simulink model "LUT_liver_pancreas_30"  (R2023b)
settings: Solver=FixedStepAuto  StartTime=0  StopTime=10.1  FixedStep=Timegap  RelTol=1e-3
model workspace (MAT data in the model file):
  T1_input = 1.34
(part 3 of 3)

== system LUT_liver_pancreas_30/If Action Subsystem6/If Action Subsystem2/If Action Subsystem9/If Action Subsystem1 ==
  In1 : Inport
  Action Port : ActionPort  ActionPortLabel=elseif( u1 >= 1.915)
  LUT 1.92RR : Lookup_n-D  NumberOfTableDimensions=1  BreakpointsForDimension1=[455.9435;504.372;599.0655;693.4809;787.3591;880.8145;973.957;1066.868;1159.606;1252.211;1344.714;1437.137;1529.495;1621.801;1714.065;1806.294;1898.493]  Table=[400;500;600;700;800;900;1000;1100;1200;1300;1400;1500;1600;1700;1800;1900;2000]  InternalRulePriority=Speed  RndMeth=Simplest
  Out1 : Outport
  wires:
  In1/1 -> LUT 1.92RR/1
  LUT 1.92RR/1 -> Out1/1

== system LUT_liver_pancreas_30/If Action Subsystem6/If Action Subsystem2/If Action Subsystem9/If Action Subsystem10 ==
  In1 : Inport
  Action Port : ActionPort  ActionPortLabel=if(u1 >= 1.995)
  LUT 2.00RR : Lookup_n-D  NumberOfTableDimensions=1  BreakpointsForDimension1=[455.5145;504.0254;598.6788;693.0105;786.7675;880.0716;973.0395;1065.758;1158.289;1250.677;1342.954;1435.143;1527.263;1619.326;1711.343;1803.322;1895.269]  Table=[400;500;600;700;800;900;1000;1100;1200;1300;1400;1500;1600;1700;1800;1900;2000]  InternalRulePriority=Speed  RndMeth=Simplest
  Out1 : Outport
  wires:
  In1/1 -> LUT 2.00RR/1
  LUT 2.00RR/1 -> Out1/1

== system LUT_liver_pancreas_30/If Action Subsystem6/If Action Subsystem2/If Action Subsystem9/If Action Subsystem11 ==
  In1 : Inport
  Action Port : ActionPort  ActionPortLabel=elseif( u1 >= 1.905)
  LUT 1.91RR : Lookup_n-D  NumberOfTableDimensions=1  BreakpointsForDimension1=[455.9998;504.4183;599.1181;693.5456;787.4408;880.9168;974.083;1067.02;1159.785;1252.42;1344.953;1437.406;1529.796;1622.134;1714.431;1806.692;1898.925]  Table=[400;500;600;700;800;900;1000;1100;1200;1300;1400;1500;1600;1700;1800;1900;2000]  InternalRulePriority=Speed  RndMeth=Simplest
  Out1 : Outport
  wires:
  In1/1 -> LUT 1.91RR/1
  LUT 1.91RR/1 -> Out1/1

== system LUT_liver_pancreas_30/If Action Subsystem6/If Action Subsystem2/If Action Subsystem9/If Action Subsystem2 ==
  In1 : Inport
  Action Port : ActionPort  ActionPortLabel=else
  LUT 1.90RR : Lookup_n-D  NumberOfTableDimensions=1  BreakpointsForDimension1=[456.0568;504.4652;599.1718;693.6118;787.5242;881.0214;974.2116;1067.175;1159.968;1252.632;1345.195;1437.68;1530.102;1622.473;1714.802;1807.097;1899.364]  Table=[400;500;600;700;800;900;1000;1100;1200;1300;1400;1500;1600;1700;1800;1900;2000]  InternalRulePriority=Speed  RndMeth=Simplest
  Out1 : Outport
  wires:
  In1/1 -> LUT 1.90RR/1
  LUT 1.90RR/1 -> Out1/1

== system LUT_liver_pancreas_30/If Action Subsystem6/If Action Subsystem2/If Action Subsystem9/If Action Subsystem3 ==
  In1 : Inport
  Action Port : ActionPort  ActionPortLabel=elseif( u1 >= 1.925)
  LUT 1.93RR : Lookup_n-D  NumberOfTableDimensions=1  BreakpointsForDimension1=[455.8877;504.3265;599.0139;693.4176;787.2793;880.7143;973.8337;1066.719;1159.43;1252.007;1344.48;1436.872;1529.199;1621.474;1713.705;1805.902;1898.068]  Table=[400;500;600;700;800;900;1000;1100;1200;1300;1400;1500;1600;1700;1800;1900;2000]  InternalRulePriority=Speed  RndMeth=Simplest
  Out1 : Outport
  wires:
  In1/1 -> LUT 1.93RR/1
  LUT 1.93RR/1 -> Out1/1

== system LUT_liver_pancreas_30/If Action Subsystem6/If Action Subsystem2/If Action Subsystem9/If Action Subsystem4 ==
  In1 : Inport
  Action Port : ActionPort  ActionPortLabel=elseif( u1 >= 1.935)
  LUT 1.94RR : Lookup_n-D  NumberOfTableDimensions=1  BreakpointsForDimension1=[455.8326;504.2816;598.9633;693.3556;787.2012;880.6164;973.7129;1066.573;1159.257;1251.806;1344.25;1436.612;1528.908;1621.152;1713.351;1805.515;1897.649]  Table=[400;500;600;700;800;900;1000;1100;1200;1300;1400;1500;1600;1700;1800;1900;2000]  InternalRulePriority=Speed  RndMeth=Simplest
  Out1 : Outport
  wires:
  In1/1 -> LUT 1.94RR/1
  LUT 1.94RR/1 -> Out1/1

== system LUT_liver_pancreas_30/If Action Subsystem6/If Action Subsystem2/If Action Subsystem9/If Action Subsystem5 ==
  In1 : Inport
  Action Port : ActionPort  ActionPortLabel=elseif( u1 >= 1.955)
  LUT 1.96RR : Lookup_n-D  NumberOfTableDimensions=1  BreakpointsForDimension1=[455.7242;504.1937;598.8648;693.2355;787.0501;880.4267;973.4788;1066.29;1158.922;1251.415;1343.802;1436.105;1528.341;1620.523;1712.66;1804.761;1896.831]  Table=[400;500;600;700;800;900;1000;1100;1200;1300;1400;1500;1600;1700;1800;1900;2000]  InternalRulePriority=Speed  RndMeth=Simplest
  Out1 : Outport
  wires:
  In1/1 -> LUT 1.96RR/1
  LUT 1.96RR/1 -> Out1/1

== system LUT_liver_pancreas_30/If Action Subsystem6/If Action Subsystem2/If Action Subsystem9/If Action Subsystem6 ==
  In1 : Inport
  Action Port : ActionPort  ActionPortLabel=elseif( u1 >= 1.945)
  LUT 1.95RR : Lookup_n-D  NumberOfTableDimensions=1  BreakpointsForDimension1=[455.7781;504.2373;598.9136;693.2949;787.1248;880.5205;973.5946;1066.431;1159.088;1251.609;1344.024;1436.356;1528.622;1620.835;1713.003;1805.135;1897.237]  Table=[400;500;600;700;800;900;1000;1100;1200;1300;1400;1500;1600;1700;1800;1900;2000]  InternalRulePriority=Speed  RndMeth=Simplest
  Out1 : Outport
  wires:
  In1/1 -> LUT 1.95RR/1
  LUT 1.95RR/1 -> Out1/1

== system LUT_liver_pancreas_30/If Action Subsystem6/If Action Subsystem2/If Action Subsystem9/If Action Subsystem7 ==
  In1 : Inport
  Action Port : ActionPort  ActionPortLabel=elseif( u1 >= 1.965)
  LUT 1.97RR : Lookup_n-D  NumberOfTableDimensions=1  BreakpointsForDimension1=[455.6709;504.1507;598.817;693.1774;786.9771;880.335;973.3654;1066.153;1158.759;1251.225;1343.584;1435.858;1528.065;1620.216;1712.323;1804.393;1896.431]  Table=[400;500;600;700;800;900;1000;1100;1200;1300;1400;1500;1600;1700;1800;1900;2000]  InternalRulePriority=Speed  RndMeth=Simplest
  Out1 : Outport
  wires:
  In1/1 -> LUT 1.97RR/1
  LUT 1.97RR/1 -> Out1/1

== system LUT_liver_pancreas_30/If Action Subsystem6/If Action Subsystem2/If Action Subsystem9/If Action Subsystem8 ==
  In1 : Inport
  Action Port : ActionPort  ActionPortLabel=elseif( u1 >= 1.975)
  LUT 1.98RR : Lookup_n-D  NumberOfTableDimensions=1  BreakpointsForDimension1=[455.6182;504.1083;598.7701;693.1206;786.9056;880.2452;973.2545;1066.019;1158.599;1251.039;1343.37;1435.616;1527.793;1619.915;1711.991;1804.03;1896.038]  Table=[400;500;600;700;800;900;1000;1100;1200;1300;1400;1500;1600;1700;1800;1900;2000]  InternalRulePriority=Speed  RndMeth=Simplest
  Out1 : Outport
  wires:
  In1/1 -> LUT 1.98RR/1
  LUT 1.98RR/1 -> Out1/1

== system LUT_liver_pancreas_30/If Action Subsystem6/If Action Subsystem2/If Action Subsystem9/If Action Subsystem9 ==
  In1 : Inport
  Action Port : ActionPort  ActionPortLabel=elseif(u1 >= 1.985)
  LUT 1.99RR : Lookup_n-D  NumberOfTableDimensions=1  BreakpointsForDimension1=[455.5661;504.0666;598.724;693.065;786.8358;880.1575;973.1458;1065.887;1158.442;1250.856;1343.16;1435.377;1527.526;1619.618;1711.664;1803.673;1895.65]  Table=[400;500;600;700;800;900;1000;1100;1200;1300;1400;1500;1600;1700;1800;1900;2000]  InternalRulePriority=Speed  RndMeth=Simplest
  Out1 : Outport
  wires:
  In1/1 -> LUT 1.99RR/1
  LUT 1.99RR/1 -> Out1/1

== system LUT_liver_pancreas_30/If Action Subsystem6/If Action Subsystem3/If Action Subsystem5/If Action Subsystem1 ==
  In1 : Inport
  Action Port : ActionPort  ActionPortLabel=elseif( u1 >= 0.615)
  LUT 0.62RR : Lookup_n-D  NumberOfTableDimensions=1  BreakpointsForDimension1=[474.416;523.9877;628.6715;734.4256;840.4801;946.6435;1052.814;1158.916;1264.875;1370.592;1475.677;1583.601;1687.634;1792.249;1896.633;2000.682;2104.35]  Table=[400;500;600;700;800;900;1000;1100;1200;1300;1400;1500;1600;1700;1800;1900;2000]  InternalRulePriority=Speed  RndMeth=Simplest
  Out1 : Outport
  wires:
  In1/1 -> LUT 0.62RR/1
  LUT 0.62RR/1 -> Out1/1

== system LUT_liver_pancreas_30/If Action Subsystem6/If Action Subsystem3/If Action Subsystem5/If Action Subsystem10 ==
  In1 : Inport
  Action Port : ActionPort  ActionPortLabel=elseif( u1 >= 0.605)
  LUT 0.61RR : Lookup_n-D  NumberOfTableDimensions=1  BreakpointsForDimension1=[474.5062;524.0083;628.793;734.7015;840.9386;947.2965;1053.661;1159.944;1266.062;1371.887;1476.748;1584.656;1689.15;1793.79;1898.122;2002.06;2105.559]  Table=[400;500;600;700;800;900;1000;1100;1200;1300;1400;1500;1600;1700;1800;1900;2000]  InternalRulePriority=Speed  RndMeth=Simplest
  Out1 : Outport
  wires:
  In1/1 -> LUT 0.61RR/1
  LUT 0.61RR/1 -> Out1/1

== system LUT_liver_pancreas_30/If Action Subsystem6/If Action Subsystem3/If Action Subsystem5/If Action Subsystem2 ==
  In1 : Inport
  Action Port : ActionPort  ActionPortLabel=else
  LUT 0.6RR : Lookup_n-D  NumberOfTableDimensions=1  BreakpointsForDimension1=[474.5798;523.9872;628.8477;734.8914;841.2953;947.8326;1054.375;1160.822;1267.075;1372.968;1477.18;1585.674;1690.376;1794.983;1899.206;2002.969;2106.229]  Table=[400;500;600;700;800;900;1000;1100;1200;1300;1400;1500;1600;1700;1800;1900;2000]  InternalRulePriority=Speed  RndMeth=Simplest
  Out1 : Outport
  wires:
  In1/1 -> LUT 0.6RR/1
  LUT 0.6RR/1 -> Out1/1

== system LUT_liver_pancreas_30/If Action Subsystem6/If Action Subsystem3/If Action Subsystem5/If Action Subsystem3 ==
  In1 : Inport
  Action Port : ActionPort  ActionPortLabel=elseif( u1 >= 0.625)
  LUT 0.63RR : Lookup_n-D  NumberOfTableDimensions=1  BreakpointsForDimension1=[474.3098;523.9296;628.4913;734.0752;839.9339;945.8908;1051.855;1157.76;1263.543;1369.122;1474.249;1582.938;1685.883;1790.418;1894.805;1998.91;2102.686]  Table=[400;500;600;700;800;900;1000;1100;1200;1300;1400;1500;1600;1700;1800;1900;2000]  InternalRulePriority=Speed  RndMeth=Simplest
  Out1 : Outport
  wires:
  In1/1 -> LUT 0.63RR/1
  LUT 0.63RR/1 -> Out1/1

== system LUT_liver_pancreas_30/If Action Subsystem6/If Action Subsystem3/If Action Subsystem5/If Action Subsystem4 ==
  In1 : Inport
  Action Port : ActionPort  ActionPortLabel=elseif( u1 >= 0.635)
  LUT 0.64RR : Lookup_n-D  NumberOfTableDimensions=1  BreakpointsForDimension1=[474.1884;523.8379;628.2596;733.6604;839.313;945.0537;1050.802;1156.498;1262.089;1367.508;1472.584;1574.402;1683.952;1788.347;1892.694;1996.809;2100.64]  Table=[400;500;600;700;800;900;1000;1100;1200;1300;1400;1500;1600;1700;1800;1900;2000]  InternalRulePriority=Speed  RndMeth=Simplest
  Out1 : Outport
  wires:
  In1/1 -> LUT 0.64RR/1
  LUT 0.64RR/1 -> Out1/1

== system LUT_liver_pancreas_30/If Action Subsystem6/If Action Subsystem3/If Action Subsystem5/If Action Subsystem5 ==
  In1 : Inport
  Action Port : ActionPort  ActionPortLabel=elseif( u1 >= 0.655)
  LUT 0.66RR : Lookup_n-D  NumberOfTableDimensions=1  BreakpointsForDimension1=[473.9037;523.5678;627.668;732.6733;837.8912;943.1792;1048.473;1153.727;1258.902;1363.951;1468.782;1572.784;1679.806;1783.66;1887.816;1991.837;2095.654]  Table=[400;500;600;700;800;900;1000;1100;1200;1300;1400;1500;1600;1700;1800;1900;2000]  InternalRulePriority=Speed  RndMeth=Simplest
  Out1 : Outport
  wires:
  In1/1 -> LUT 0.66RR/1
  LUT 0.66RR/1 -> Out1/1

== system LUT_liver_pancreas_30/If Action Subsystem6/If Action Subsystem3/If Action Subsystem5/If Action Subsystem6 ==
  In1 : Inport
  Action Port : ActionPort  ActionPortLabel=elseif( u1 >= 0.645)
  LUT 0.65RR : Lookup_n-D  NumberOfTableDimensions=1  BreakpointsForDimension1=[474.0528;523.7162;627.9832;733.1903;838.6287;944.1458;1049.669;1155.148;1260.536;1365.777;1470.748;1574.214;1681.9;1786.081;1890.35;1994.435;2098.278]  Table=[400;500;600;700;800;900;1000;1100;1200;1300;1400;1500;1600;1700;1800;1900;2000]  InternalRulePriority=Speed  RndMeth=Simplest
  Out1 : Outport
  wires:
  In1/1 -> LUT 0.65RR/1
  LUT 0.65RR/1 -> Out1/1

== system LUT_liver_pancreas_30/If Action Subsystem6/If Action Subsystem3/If Action Subsystem5/If Action Subsystem7 ==
  In1 : Inport
  Action Port : ActionPort  ActionPortLabel=elseif( u1 >= 0.665)
  LUT 0.67RR : Lookup_n-D  NumberOfTableDimensions=1  BreakpointsForDimension1=[473.7423;523.3958;627.3195;732.1167;837.1095;942.1646;1047.224;1152.249;1257.204;1362.051;1466.718;1570.857;1677.824;1781.119;1885.13;1989.059;2092.817]  Table=[400;500;600;700;800;900;1000;1100;1200;1300;1400;1500;1600;1700;1800;1900;2000]  InternalRulePriority=Speed  RndMeth=Simplest
  Out1 : Outport
  wires:
  In1/1 -> LUT 0.67RR/1
  LUT 0.67RR/1 -> Out1/1

== system LUT_liver_pancreas_30/If Action Subsystem6/If Action Subsystem3/If Action Subsystem5/If Action Subsystem8 ==
  In1 : Inport
  Action Port : ActionPort  ActionPortLabel=elseif(u1 >= 0.675)
  LUT 0.68RR : Lookup_n-D  NumberOfTableDimensions=1  BreakpointsForDimension1=[473.5695;523.203;626.9426;731.527;836.2917;941.1114;1045.934;1150.726;1255.457;1360.093;1464.579;1568.697;1676.389;1778.492;1882.325;1986.137;2089.81]  Table=[400;500;600;700;800;900;1000;1100;1200;1300;1400;1500;1600;1700;1800;1900;2000]  InternalRulePriority=Speed  RndMeth=Simplest
  Out1 : Outport
  wires:
  In1/1 -> LUT 0.68RR/1
  LUT 0.68RR/1 -> Out1/1

== system LUT_liver_pancreas_30/If Action Subsystem6/If Action Subsystem3/If Action Subsystem5/If Action Subsystem9 ==
  In1 : Inport
  Action Port : ActionPort  ActionPortLabel=if(u1 >= 0.685)
  LUT 0.69RR : Lookup_n-D  NumberOfTableDimensions=1  BreakpointsForDimension1=[473.3863;522.992;626.5416;730.9101;835.4449;940.028;1044.613;1149.17;1253.672;1358.092;1462.386;1566.406;1667.106;1775.814;1879.429;1983.102;2086.667]  Table=[400;500;600;700;800;900;1000;1100;1200;1300;1400;1500;1600;1700;1800;1900;2000]  InternalRulePriority=Speed  RndMeth=Simplest
  Out1 : Outport
  wires:
  In1/1 -> LUT 0.69RR/1
  LUT 0.69RR/1 -> Out1/1

== system LUT_liver_pancreas_30/If Action Subsystem6/If Action Subsystem3/If Action Subsystem6/If Action Subsystem1 ==
  In1 : Inport
  Action Port : ActionPort  ActionPortLabel=elseif( u1 >= 0.515)
  LUT 0.52RR : Lookup_n-D  NumberOfTableDimensions=1  BreakpointsForDimension1=[474.5762;521.7393;625.6496;731.5358;838.1904;945.1164;1051.969;1158.437;1263.932;1371.564;1475.254;1578.61;1680.944;1782.085;1881.929;1980.397;2077.433]  Table=[400;500;600;700;800;900;1000;1100;1200;1300;1400;1500;1600;1700;1800;1900;2000]  InternalRulePriority=Speed  RndMeth=Simplest
  Out1 : Outport
  wires:
  In1/1 -> LUT 0.52RR/1
  LUT 0.52RR/1 -> Out1/1

== system LUT_liver_pancreas_30/If Action Subsystem6/If Action Subsystem3/If Action Subsystem6/If Action Subsystem10 ==
  In1 : Inport
  Action Port : ActionPort  ActionPortLabel=elseif( u1 >= 0.505)
  LUT 0.51RR : Lookup_n-D  NumberOfTableDimensions=1  BreakpointsForDimension1=[474.5205;521.1183;624.6064;730.2245;836.688;943.4438;1050.1;1156.292;1261.116;1368.302;1471.738;1574.405;1675.861;1775.944;1874.546;1971.588;2067.015]  Table=[400;500;600;700;800;900;1000;1100;1200;1300;1400;1500;1600;1700;1800;1900;2000]  InternalRulePriority=Speed  RndMeth=Simplest
  Out1 : Outport
  wires:
  In1/1 -> LUT 0.51RR/1
  LUT 0.51RR/1 -> Out1/1

== system LUT_liver_pancreas_30/If Action Subsystem6/If Action Subsystem3/If Action Subsystem6/If Action Subsystem2 ==
  In1 : Inport
  Action Port : ActionPort  ActionPortLabel=else
  LUT 0.50RR : Lookup_n-D  NumberOfTableDimensions=1  BreakpointsForDimension1=[474.463;520.4034;623.3708;728.6386;834.8363;941.3471;1047.726;1153.541;1257.231;1364.382;1467.272;1569.079;1669.469;1768.286;1865.417;1960.783;2054.337]  Table=[400;500;600;700;800;900;1000;1100;1200;1300;1400;1500;1600;1700;1800;1900;2000]  InternalRulePriority=Speed  RndMeth=Simplest
  Out1 : Outport
  wires:
  In1/1 -> LUT 0.50RR/1
  LUT 0.50RR/1 -> Out1/1

== system LUT_liver_pancreas_30/If Action Subsystem6/If Action Subsystem3/If Action Subsystem6/If Action Subsystem3 ==
  In1 : Inport
  Action Port : ActionPort  ActionPortLabel=elseif( u1 >= 0.525)
  LUT 0.53RR : Lookup_n-D  NumberOfTableDimensions=1  BreakpointsForDimension1=[474.6253;522.2718;626.5165;732.598;839.3776;946.4084;1053.386;1160.044;1265.963;1365.661;1477.938;1581.826;1684.873;1786.888;1887.77;1987.443;2085.85]  Table=[400;500;600;700;800;900;1000;1100;1200;1300;1400;1500;1600;1700;1800;1900;2000]  InternalRulePriority=Speed  RndMeth=Simplest
  Out1 : Outport
  wires:
  In1/1 -> LUT 0.53RR/1
  LUT 0.53RR/1 -> Out1/1

== system LUT_liver_pancreas_30/If Action Subsystem6/If Action Subsystem3/If Action Subsystem6/If Action Subsystem4 ==
  In1 : Inport
  Action Port : ActionPort  ActionPortLabel=elseif( u1 >= 0.535)
  LUT 0.54RR : Lookup_n-D  NumberOfTableDimensions=1  BreakpointsForDimension1=[474.6644;522.7214;627.2226;733.4352;840.282;947.3604;1054.402;1161.177;1267.368;1369.963;1479.904;1584.175;1687.789;1790.518;1892.259;1992.94;2092.504]  Table=[400;500;600;700;800;900;1000;1100;1200;1300;1400;1500;1600;1700;1800;1900;2000]  InternalRulePriority=Speed  RndMeth=Simplest
  Out1 : Outport
  wires:
  In1/1 -> LUT 0.54RR/1
  LUT 0.54RR/1 -> Out1/1

== system LUT_liver_pancreas_30/If Action Subsystem6/If Action Subsystem3/If Action Subsystem6/If Action Subsystem5 ==
  In1 : Inport
  Action Port : ActionPort  ActionPortLabel=elseif( u1 >= 0.555)
  LUT 0.56RR : Lookup_n-D  NumberOfTableDimensions=1  BreakpointsForDimension1=[474.702;523.3943;628.2103;734.5232;841.36;948.3917;1055.409;1162.239;1268.68;1373.96;1482.145;1586.707;1691.087;1794.838;1897.845;2000.041;2101.376]  Table=[400;500;600;700;800;900;1000;1100;1200;1300;1400;1500;1600;1700;1800;1900;2000]  InternalRulePriority=Speed  RndMeth=Simplest
  Out1 : Outport
  wires:
  In1/1 -> LUT 0.56RR/1
  LUT 0.56RR/1 -> Out1/1

== system LUT_liver_pancreas_30/If Action Subsystem6/If Action Subsystem3/If Action Subsystem6/If Action Subsystem6 ==
  In1 : Inport
  Action Port : ActionPort  ActionPortLabel=elseif( u1 >= 0.545)
  LUT 0.55RR : Lookup_n-D  NumberOfTableDimensions=1  BreakpointsForDimension1=[474.6906;523.0937;627.7826;734.0699;840.9336;948.01;1055.062;1161.891;1268.247;1372.673;1481.264;1585.769;1689.822;1793.124;1895.566;1997.081;2097.613]  Table=[400;500;600;700;800;900;1000;1100;1200;1300;1400;1500;1600;1700;1800;1900;2000]  InternalRulePriority=Speed  RndMeth=Simplest
  Out1 : Outport
  wires:
  In1/1 -> LUT 0.55RR/1
  LUT 0.55RR/1 -> Out1/1

== system LUT_liver_pancreas_30/If Action Subsystem6/If Action Subsystem3/If Action Subsystem6/If Action Subsystem7 ==
  In1 : Inport
  Action Port : ActionPort  ActionPortLabel=elseif( u1 >= 0.565)
  LUT 0.57RR : Lookup_n-D  NumberOfTableDimensions=1  BreakpointsForDimension1=[474.6972;523.6287;628.519;734.8148;841.587;948.5373;1055.481;1162.266;1268.728;1374.402;1482.732;1587.083;1691.687;1795.78;1899.232;2001.978;2103.969]  Table=[400;500;600;700;800;900;1000;1100;1200;1300;1400;1500;1600;1700;1800;1900;2000]  InternalRulePriority=Speed  RndMeth=Simplest
  Out1 : Outport
  wires:
  In1/1 -> LUT 0.57RR/1
  LUT 0.57RR/1 -> Out1/1

== system LUT_liver_pancreas_30/If Action Subsystem6/If Action Subsystem3/If Action Subsystem6/If Action Subsystem8 ==
  In1 : Inport
  Action Port : ActionPort  ActionPortLabel=elseif(u1 >= 0.575)
  LUT 0.58RR : Lookup_n-D  NumberOfTableDimensions=1  BreakpointsForDimension1=[474.6754;523.8022;628.7207;734.9626;841.638;948.4755;1055.312;1162.015;1268.446;1374.298;1473.533;1586.981;1691.715;1796.057;1899.852;2003.032;2105.551]  Table=[400;500;600;700;800;900;1000;1100;1200;1300;1400;1500;1600;1700;1800;1900;2000]  InternalRulePriority=Speed  RndMeth=Simplest
  Out1 : Outport
  wires:
  In1/1 -> LUT 0.58RR/1
  LUT 0.58RR/1 -> Out1/1

== system LUT_liver_pancreas_30/If Action Subsystem6/If Action Subsystem3/If Action Subsystem6/If Action Subsystem9 ==
  In1 : Inport
  Action Port : ActionPort  ActionPortLabel=if(u1 >= 0.585)
  LUT 0.59RR : Lookup_n-D  NumberOfTableDimensions=1  BreakpointsForDimension1=[474.6363;523.9201;628.8268;734.9831;841.5343;948.2328;1054.934;1161.522;1267.881;1373.792;1476.295;1586.484;1691.253;1795.763;1899.811;2003.325;2106.263]  Table=[400;500;600;700;800;900;1000;1100;1200;1300;1400;1500;1600;1700;1800;1900;2000]  InternalRulePriority=Speed  RndMeth=Simplest
  Out1 : Outport
  wires:
  In1/1 -> LUT 0.59RR/1
  LUT 0.59RR/1 -> Out1/1

== system LUT_liver_pancreas_30/If Action Subsystem6/If Action Subsystem3/If Action Subsystem7/If Action Subsystem1 ==
  In1 : Inport
  Action Port : ActionPort  ActionPortLabel=elseif( u1 >= 0.715)
  LUT 0.72RR : Lookup_n-D  NumberOfTableDimensions=1  BreakpointsForDimension1=[472.7837;522.2728;625.232;728.945;832.7895;936.6649;1040.537;1144.387;1248.198;1351.952;1455.625;1559.161;1662.226;1768.021;1870.441;1973.584;2076.721]  Table=[400;500;600;700;800;900;1000;1100;1200;1300;1400;1500;1600;1700;1800;1900;2000]  InternalRulePriority=Speed  RndMeth=Simplest
  Out1 : Outport
  wires:
  In1/1 -> LUT 0.72RR/1
  LUT 0.72RR/1 -> Out1/1

== system LUT_liver_pancreas_30/If Action Subsystem6/If Action Subsystem3/If Action Subsystem7/If Action Subsystem10 ==
  In1 : Inport
  Action Port : ActionPort  ActionPortLabel=elseif( u1 >= 0.705)
  LUT 0.71RR : Lookup_n-D  NumberOfTableDimensions=1  BreakpointsForDimension1=[472.9925;522.5248;625.683;729.6147;833.6886;937.7988;1041.908;1145.992;1250.034;1354.012;1457.896;1561.613;1664.565;1770.484;1873.466;1976.804;2080.098]  Table=[400;500;600;700;800;900;1000;1100;1200;1300;1400;1500;1600;1700;1800;1900;2000]  InternalRulePriority=Speed  RndMeth=Simplest
  Out1 : Outport
  wires:
  In1/1 -> LUT 0.71RR/1
  LUT 0.71RR/1 -> Out1/1

== system LUT_liver_pancreas_30/If Action Subsystem6/If Action Subsystem3/If Action Subsystem7/If Action Subsystem2 ==
  In1 : Inport
  Action Port : ActionPort  ActionPortLabel=else
  LUT 0.70RR : Lookup_n-D  NumberOfTableDimensions=1  BreakpointsForDimension1=[473.1936;522.7652;626.1206;730.2711;834.5754;938.9217;1043.268;1147.589;1251.861;1356.062;1460.154;1564.034;1666.473;1773.124;1876.469;1979.983;2083.421]  Table=[400;500;600;700;800;900;1000;1100;1200;1300;1400;1500;1600;1700;1800;1900;2000]  InternalRulePriority=Speed  RndMeth=Simplest
  Out1 : Outport
  wires:
  In1/1 -> LUT 0.70RR/1
  LUT 0.70RR/1 -> Out1/1

== system LUT_liver_pancreas_30/If Action Subsystem6/If Action Subsystem3/If Action Subsystem7/If Action Subsystem3 ==
  In1 : Inport
  Action Port : ActionPort  ActionPortLabel=elseif( u1 >= 0.725)
  LUT 0.73RR : Lookup_n-D  NumberOfTableDimensions=1  BreakpointsForDimension1=[472.5683;522.011;624.7704;728.2654;831.8822;935.5249;1039.163;1142.779;1246.36;1349.89;1453.35;1556.696;1659.72;1766.121;1867.415;1970.342;2073.311]  Table=[400;500;600;700;800;900;1000;1100;1200;1300;1400;1500;1600;1700;1800;1900;2000]  InternalRulePriority=Speed  RndMeth=Simplest
  Out1 : Outport
  wires:
  In1/1 -> LUT 0.73RR/1
  LUT 0.73RR/1 -> Out1/1

== system LUT_liver_pancreas_30/If Action Subsystem6/If Action Subsystem3/If Action Subsystem7/If Action Subsystem4 ==
  In1 : Inport
  Action Port : ActionPort  ActionPortLabel=elseif( u1 >= 0.735)
  LUT 0.74RR : Lookup_n-D  NumberOfTableDimensions=1  BreakpointsForDimension1=[472.3471;521.741;624.3008;727.5792;830.9705;934.3829;1037.789;1141.174;1244.526;1347.833;1451.079;1554.227;1657.143;1766.068;1864.407;1967.093;2069.882]  Table=[400;500;600;700;800;900;1000;1100;1200;1300;1400;1500;1600;1700;1800;1900;2000]  InternalRulePriority=Speed  RndMeth=Simplest
  Out1 : Outport
  wires:
  In1/1 -> LUT 0.74RR/1
  LUT 0.74RR/1 -> Out1/1

== system LUT_liver_pancreas_30/If Action Subsystem6/If Action Subsystem3/If Action Subsystem7/If Action Subsystem5 ==
  In1 : Inport
  Action Port : ActionPort  ActionPortLabel=elseif( u1 >= 0.755)
  LUT 0.76RR : Lookup_n-D  NumberOfTableDimensions=1  BreakpointsForDimension1=[471.8903;521.182;623.3456;726.1977;829.1462;932.1073;1035.058;1137.989;1240.892;1343.757;1446.574;1549.319;1651.925;1753.767;1858.578;1960.627;2063.029]  Table=[400;500;600;700;800;900;1000;1100;1200;1300;1400;1500;1600;1700;1800;1900;2000]  InternalRulePriority=Speed  RndMeth=Simplest
  Out1 : Outport
  wires:
  In1/1 -> LUT 0.76RR/1
  LUT 0.76RR/1 -> Out1/1

== system LUT_liver_pancreas_30/If Action Subsystem6/If Action Subsystem3/If Action Subsystem7/If Action Subsystem6 ==
  In1 : Inport
  Action Port : ActionPort  ActionPortLabel=elseif( u1 >= 0.745)
  LUT 0.75RR : Lookup_n-D  NumberOfTableDimensions=1  BreakpointsForDimension1=[472.1208;521.4642;623.8252;726.8892;830.0576;933.2427;1036.42;1139.576;1242.702;1345.787;1448.818;1551.766;1654.537;1755.796;1861.447;1963.851;2066.451]  Table=[400;500;600;700;800;900;1000;1100;1200;1300;1400;1500;1600;1700;1800;1900;2000]  InternalRulePriority=Speed  RndMeth=Simplest
  Out1 : Outport
  wires:
  In1/1 -> LUT 0.75RR/1
  LUT 0.75RR/1 -> Out1/1

== system LUT_liver_pancreas_30/If Action Subsystem6/If Action Subsystem3/If Action Subsystem7/If Action Subsystem7 ==
  In1 : Inport
  Action Port : ActionPort  ActionPortLabel=elseif( u1 >= 0.765)
  LUT 0.77RR : Lookup_n-D  NumberOfTableDimensions=1  BreakpointsForDimension1=[471.6561;520.8957;622.8639;725.5068;828.2389;930.9794;1033.708;1136.417;1239.099;1341.746;1444.35;1546.892;1649.322;1751.296;1855.899;1957.433;2059.627]  Table=[400;500;600;700;800;900;1000;1100;1200;1300;1400;1500;1600;1700;1800;1900;2000]  InternalRulePriority=Speed  RndMeth=Simplest
  Out1 : Outport
  wires:
  In1/1 -> LUT 0.77RR/1
  LUT 0.77RR/1 -> Out1/1

== system LUT_liver_pancreas_30/If Action Subsystem6/If Action Subsystem3/If Action Subsystem7/If Action Subsystem8 ==
  In1 : Inport
  Action Port : ActionPort  ActionPortLabel=elseif(u1 >= 0.775)
  LUT 0.78RR : Lookup_n-D  NumberOfTableDimensions=1  BreakpointsForDimension1=[471.4191;520.6062;622.3814;724.8183;827.3375;929.8614;1032.372;1134.862;1237.326;1339.759;1442.152;1544.491;1646.737;1748.681;1853.716;1954.282;2056.254]  Table=[400;500;600;700;800;900;1000;1100;1200;1300;1400;1500;1600;1700;1800;1900;2000]  InternalRulePriority=Speed  RndMeth=Simplest
  Out1 : Outport
  wires:
  In1/1 -> LUT 0.78RR/1
  LUT 0.78RR/1 -> Out1/1

== system LUT_liver_pancreas_30/If Action Subsystem6/If Action Subsystem3/If Action Subsystem7/If Action Subsystem9 ==
  In1 : Inport
  Action Port : ActionPort  ActionPortLabel=if(u1 >= 0.785)
  LUT 0.79RR : Lookup_n-D  NumberOfTableDimensions=1  BreakpointsForDimension1=[471.1797;520.3146;621.8995;724.1339;826.444;928.7551;1031.051;1133.326;1235.576;1337.797;1439.982;1542.119;1644.179;1746.023;1853.155;1951.185;2052.917]  Table=[400;500;600;700;800;900;1000;1100;1200;1300;1400;1500;1600;1700;1800;1900;2000]  InternalRulePriority=Speed  RndMeth=Simplest
  Out1 : Outport
  wires:
  In1/1 -> LUT 0.79RR/1
  LUT 0.79RR/1 -> Out1/1

== system LUT_liver_pancreas_30/If Action Subsystem6/If Action Subsystem3/If Action Subsystem8/If Action Subsystem1 ==
  In1 : Inport
  Action Port : ActionPort  ActionPortLabel=elseif( u1 >= 0.815)
  LUT 0.82RR : Lookup_n-D  NumberOfTableDimensions=1  BreakpointsForDimension1=[470.4531;519.4351;620.4683;722.1174;823.8242;925.5214;1027.198;1128.852;1230.483;1332.089;1433.666;1535.209;1636.702;1738.096;1839.013;1942.508;2043.189]  Table=[400;500;600;700;800;900;1000;1100;1200;1300;1400;1500;1600;1700;1800;1900;2000]  InternalRulePriority=Speed  RndMeth=Simplest
  Out1 : Outport
  wires:
  In1/1 -> LUT 0.82RR/1
  LUT 0.82RR/1 -> Out1/1

== system LUT_liver_pancreas_30/If Action Subsystem6/If Action Subsystem3/If Action Subsystem8/If Action Subsystem10 ==
  In1 : Inport
  Action Port : ActionPort  ActionPortLabel=elseif( u1 >= 0.805)
  LUT 0.81RR : Lookup_n-D  NumberOfTableDimensions=1  BreakpointsForDimension1=[470.6962;519.7283;620.942;722.7824;824.6862;926.5838;1028.463;1130.32;1232.153;1333.96;1435.737;1537.476;1639.158;1740.714;1841.442;1945.245;2046.378]  Table=[400;500;600;700;800;900;1000;1100;1200;1300;1400;1500;1600;1700;1800;1900;2000]  InternalRulePriority=Speed  RndMeth=Simplest
  Out1 : Outport
  wires:
  In1/1 -> LUT 0.81RR/1
  LUT 0.81RR/1 -> Out1/1

== system LUT_liver_pancreas_30/If Action Subsystem6/If Action Subsystem3/If Action Subsystem8/If Action Subsystem2 ==
  In1 : Inport
  Action Port : ActionPort  ActionPortLabel=else
  LUT 0.80RR : Lookup_n-D  NumberOfTableDimensions=1  BreakpointsForDimension1=[470.9386;520.0217;621.4194;723.4549;825.5598;927.6621;1029.747;1131.811;1233.851;1335.864;1437.843;1539.78;1641.651;1743.36;1843.325;1948.162;2049.623]  Table=[400;500;600;700;800;900;1000;1100;1200;1300;1400;1500;1600;1700;1800;1900;2000]  InternalRulePriority=Speed  RndMeth=Simplest
  Out1 : Outport
  wires:
  In1/1 -> LUT 0.80RR/1
  LUT 0.80RR/1 -> Out1/1

== system LUT_liver_pancreas_30/If Action Subsystem6/If Action Subsystem3/If Action Subsystem8/If Action Subsystem3 ==
  In1 : Inport
  Action Port : ActionPort  ActionPortLabel=elseif( u1 >= 0.825)
  LUT 0.83RR : Lookup_n-D  NumberOfTableDimensions=1  BreakpointsForDimension1=[470.2097;519.1426;619.999;721.4608;822.9747;924.4756;1025.954;1127.409;1228.841;1330.25;1431.631;1532.981;1634.287;1735.512;1836.429;1940.169;2040.062]  Table=[400;500;600;700;800;900;1000;1100;1200;1300;1400;1500;1600;1700;1800;1900;2000]  InternalRulePriority=Speed  RndMeth=Simplest
  Out1 : Outport
  wires:
  In1/1 -> LUT 0.83RR/1
  LUT 0.83RR/1 -> Out1/1

== system LUT_liver_pancreas_30/If Action Subsystem6/If Action Subsystem3/If Action Subsystem8/If Action Subsystem4 ==
  In1 : Inport
  Action Port : ActionPort  ActionPortLabel=elseif( u1 >= 0.835)
  LUT 0.84RR : Lookup_n-D  NumberOfTableDimensions=1  BreakpointsForDimension1=[469.9663;518.8514;619.5346;720.8133;822.1384;923.4473;1024.732;1125.992;1227.23;1328.444;1429.633;1530.793;1631.914;1732.967;1833.806;1939.076;2037.006]  Table=[400;500;600;700;800;900;1000;1100;1200;1300;1400;1500;1600;1700;1800;1900;2000]  InternalRulePriority=Speed  RndMeth=Simplest
  Out1 : Outport
  wires:
  In1/1 -> LUT 0.84RR/1
  LUT 0.84RR/1 -> Out1/1

== system LUT_liver_pancreas_30/If Action Subsystem6/If Action Subsystem3/If Action Subsystem8/If Action Subsystem5 ==
  In1 : Inport
  Action Port : ActionPort  ActionPortLabel=elseif( u1 >= 0.855)
  LUT 0.86RR : Lookup_n-D  NumberOfTableDimensions=1  BreakpointsForDimension1=[469.4814;518.2747;618.6232;719.5475;820.5076;921.4451;1022.355;1123.238;1224.098;1324.935;1425.75;1526.54;1627.298;1728.006;1828.594;1928.211;2031.167]  Table=[400;500;600;700;800;900;1000;1100;1200;1300;1400;1500;1600;1700;1800;1900;2000]  InternalRulePriority=Speed  RndMeth=Simplest
  Out1 : Outport
  wires:
  In1/1 -> LUT 0.86RR/1
  LUT 0.86RR/1 -> Out1/1

== system LUT_liver_pancreas_30/If Action Subsystem6/If Action Subsystem3/If Action Subsystem8/If Action Subsystem6 ==
  In1 : Inport
  Action Port : ActionPort  ActionPortLabel=elseif( u1 >= 0.845)
  LUT 0.85RR : Lookup_n-D  NumberOfTableDimensions=1  BreakpointsForDimension1=[469.7235;518.5619;619.0759;720.1753;821.3159;922.437;1023.532;1124.602;1225.649;1326.672;1427.673;1528.646;1629.584;1730.465;1831.188;1941.317;2034.033]  Table=[400;500;600;700;800;900;1000;1100;1200;1300;1400;1500;1600;1700;1800;1900;2000]  InternalRulePriority=Speed  RndMeth=Simplest
  Out1 : Outport
  wires:
  In1/1 -> LUT 0.85RR/1
  LUT 0.85RR/1 -> Out1/1

== system LUT_liver_pancreas_30/If Action Subsystem6/If Action Subsystem3/If Action Subsystem8/If Action Subsystem7 ==
  In1 : Inport
  Action Port : ActionPort  ActionPortLabel=elseif( u1 >= 0.865)
  LUT 0.87RR : Lookup_n-D  NumberOfTableDimensions=1  BreakpointsForDimension1=[469.2404;517.99;618.1768;718.93;819.7139;920.4719;1021.2;1121.901;1222.578;1323.233;1423.866;1524.475;1625.056;1725.593;1826.035;1925.946;2028.461]  Table=[400;500;600;700;800;900;1000;1100;1200;1300;1400;1500;1600;1700;1800;1900;2000]  InternalRulePriority=Speed  RndMeth=Simplest
  Out1 : Outport
  wires:
  In1/1 -> LUT 0.87RR/1
  LUT 0.87RR/1 -> Out1/1

== system LUT_liver_pancreas_30/If Action Subsystem6/If Action Subsystem3/If Action Subsystem8/If Action Subsystem8 ==
  In1 : Inport
  Action Port : ActionPort  ActionPortLabel=elseif(u1 >= 0.875)
  LUT 0.88RR : Lookup_n-D  NumberOfTableDimensions=1  BreakpointsForDimension1=[469.0007;517.7081;617.7372;718.3234;818.935;919.5176;1020.068;1120.591;1221.089;1321.565;1422.02;1522.452;1622.858;1723.226;1823.517;1923.475;2026.064]  Table=[400;500;600;700;800;900;1000;1100;1200;1300;1400;1500;1600;1700;1800;1900;2000]  InternalRulePriority=Speed  RndMeth=Simplest
  Out1 : Outport
  wires:
  In1/1 -> LUT 0.88RR/1
  LUT 0.88RR/1 -> Out1/1

== system LUT_liver_pancreas_30/If Action Subsystem6/If Action Subsystem3/If Action Subsystem8/If Action Subsystem9 ==
  In1 : Inport
  Action Port : ActionPort  ActionPortLabel=if(u1 >= 0.885)
  LUT 0.89RR : Lookup_n-D  NumberOfTableDimensions=1  BreakpointsForDimension1=[468.7627;517.4293;617.3046;717.7277;818.171;918.5823;1018.96;1119.308;1219.631;1319.932;1420.212;1520.471;1620.705;1720.905;1821.042;1920.953;2024.538]  Table=[400;500;600;700;800;900;1000;1100;1200;1300;1400;1500;1600;1700;1800;1900;2000]  InternalRulePriority=Speed  RndMeth=Simplest
  Out1 : Outport
  wires:
  In1/1 -> LUT 0.89RR/1
  LUT 0.89RR/1 -> Out1/1

== system LUT_liver_pancreas_30/If Action Subsystem6/If Action Subsystem3/If Action Subsystem9/If Action Subsystem1 ==
  In1 : Inport
  Action Port : ActionPort  ActionPortLabel=elseif( u1 >= 0.915)
  LUT 0.92RR : Lookup_n-D  NumberOfTableDimensions=1  BreakpointsForDimension1=[468.06;516.6138;616.0504;716.0075;815.9697;915.8904;1015.771;1115.619;1215.44;1315.238;1415.016;1514.774;1614.512;1714.224;1813.897;1913.473;2012.422]  Table=[400;500;600;700;800;900;1000;1100;1200;1300;1400;1500;1600;1700;1800;1900;2000]  InternalRulePriority=Speed  RndMeth=Simplest
  Out1 : Outport
  wires:
  In1/1 -> LUT 0.92RR/1
  LUT 0.92RR/1 -> Out1/1

== system LUT_liver_pancreas_30/If Action Subsystem6/If Action Subsystem3/If Action Subsystem9/If Action Subsystem10 ==
  In1 : Inport
  Action Port : ActionPort  ActionPortLabel=elseif( u1 >= 0.905)
  LUT 0.91RR : Lookup_n-D  NumberOfTableDimensions=1  BreakpointsForDimension1=[468.2921;516.882;616.4611;716.5697;816.6884;916.7688;1016.811;1116.822;1216.807;1316.769;1416.711;1516.632;1616.532;1716.405;1816.231;1915.935;2014.415]  Table=[400;500;600;700;800;900;1000;1100;1200;1300;1400;1500;1600;1700;1800;1900;2000]  InternalRulePriority=Speed  RndMeth=Simplest
  Out1 : Outport
  wires:
  In1/1 -> LUT 0.91RR/1
  LUT 0.91RR/1 -> Out1/1

== system LUT_liver_pancreas_30/If Action Subsystem6/If Action Subsystem3/If Action Subsystem9/If Action Subsystem2 ==
  In1 : Inport
  Action Port : ActionPort  ActionPortLabel=else
  LUT 0.90RR : Lookup_n-D  NumberOfTableDimensions=1  BreakpointsForDimension1=[468.5264;517.1539;616.8792;717.1431;817.4222;917.6661;1017.874;1118.052;1218.204;1318.333;1418.443;1518.531;1618.597;1718.632;1818.613;1918.432;2025.833]  Table=[400;500;600;700;800;900;1000;1100;1200;1300;1400;1500;1600;1700;1800;1900;2000]  InternalRulePriority=Speed  RndMeth=Simplest
  Out1 : Outport
  wires:
  In1/1 -> LUT 0.90RR/1
  LUT 0.90RR/1 -> Out1/1

== system LUT_liver_pancreas_30/If Action Subsystem6/If Action Subsystem3/If Action Subsystem9/If Action Subsystem3 ==
  In1 : Inport
  Action Port : ActionPort  ActionPortLabel=elseif( u1 >= 0.925)
  LUT 0.93RR : Lookup_n-D  NumberOfTableDimensions=1  BreakpointsForDimension1=[467.8302;516.3494;615.6473;715.4567;815.2661;915.0307;1014.753;1114.442;1214.102;1313.74;1413.357;1512.956;1612.534;1712.089;1811.609;1911.052;2010.117]  Table=[400;500;600;700;800;900;1000;1100;1200;1300;1400;1500;1600;1700;1800;1900;2000]  InternalRulePriority=Speed  RndMeth=Simplest
  Out1 : Outport
  wires:
  In1/1 -> LUT 0.93RR/1
  LUT 0.93RR/1 -> Out1/1

== system LUT_liver_pancreas_30/If Action Subsystem6/If Action Subsystem3/If Action Subsystem9/If Action Subsystem4 ==
  In1 : Inport
  Action Port : ActionPort  ActionPortLabel=elseif( u1 >= 0.935)
  LUT 0.94RR : Lookup_n-D  NumberOfTableDimensions=1  BreakpointsForDimension1=[467.6029;516.089;615.2518;714.9171;814.5773;914.1896;1013.758;1113.29;1212.794;1312.275;1411.735;1511.177;1610.599;1710;1809.369;1908.675;2007.731]  Table=[400;500;600;700;800;900;1000;1100;1200;1300;1400;1500;1600;1700;1800;1900;2000]  InternalRulePriority=Speed  RndMeth=Simplest
  Out1 : Outport
  wires:
  In1/1 -> LUT 0.94RR/1
  LUT 0.94RR/1 -> Out1/1

== system LUT_liver_pancreas_30/If Action Subsystem6/If Action Subsystem3/If Action Subsystem9/If Action Subsystem5 ==
  In1 : Inport
  Action Port : ActionPort  ActionPortLabel=elseif( u1 >= 0.955)
  LUT 0.96RR : Lookup_n-D  NumberOfTableDimensions=1  BreakpointsForDimension1=[467.1559;515.5802;614.4835;713.8713;813.2439;912.5621;1011.832;1111.063;1210.264;1309.441;1408.597;1507.735;1606.854;1705.954;1805.028;1904.058;2002.955]  Table=[400;500;600;700;800;900;1000;1100;1200;1300;1400;1500;1600;1700;1800;1900;2000]  InternalRulePriority=Speed  RndMeth=Simplest
  Out1 : Outport
  wires:
  In1/1 -> LUT 0.96RR/1
  LUT 0.96RR/1 -> Out1/1

== system LUT_liver_pancreas_30/If Action Subsystem6/If Action Subsystem3/If Action Subsystem9/If Action Subsystem6 ==
  In1 : Inport
  Action Port : ActionPort  ActionPortLabel=elseif( u1 >= 0.945)
  LUT 0.95RR : Lookup_n-D  NumberOfTableDimensions=1  BreakpointsForDimension1=[467.378;515.8325;614.8638;714.3886;813.9033;913.3668;1012.784;1112.164;1211.515;1310.842;1410.149;1509.437;1608.706;1707.955;1807.176;1906.343;2005.334]  Table=[400;500;600;700;800;900;1000;1100;1200;1300;1400;1500;1600;1700;1800;1900;2000]  InternalRulePriority=Speed  RndMeth=Simplest
  Out1 : Outport
  wires:
  In1/1 -> LUT 0.95RR/1
  LUT 0.95RR/1 -> Out1/1

== system LUT_liver_pancreas_30/If Action Subsystem6/If Action Subsystem3/If Action Subsystem9/If Action Subsystem7 ==
  In1 : Inport
  Action Port : ActionPort  ActionPortLabel=elseif( u1 >= 0.965)
  LUT 0.97RR : Lookup_n-D  NumberOfTableDimensions=1  BreakpointsForDimension1=[466.9364;515.332;614.1107;713.365;812.5989;911.7751;1010.901;1109.987;1209.041;1308.071;1407.08;1506.07;1605.042;1703.996;1802.927;1901.818;2000.608]  Table=[400;500;600;700;800;900;1000;1100;1200;1300;1400;1500;1600;1700;1800;1900;2000]  InternalRulePriority=Speed  RndMeth=Simplest
  Out1 : Outport
  wires:
  In1/1 -> LUT 0.97RR/1
  LUT 0.97RR/1 -> Out1/1

== system LUT_liver_pancreas_30/If Action Subsystem6/If Action Subsystem3/If Action Subsystem9/If Action Subsystem8 ==
  In1 : Inport
  Action Port : ActionPort  ActionPortLabel=elseif(u1 >= 0.975)
  LUT 0.98RR : Lookup_n-D  NumberOfTableDimensions=1  BreakpointsForDimension1=[466.7197;515.088;613.7454;712.8695;811.9681;911.0057;1009.99;1108.934;1207.845;1306.731;1405.596;1504.442;1603.27;1702.081;1800.87;1899.624;1998.299]  Table=[400;500;600;700;800;900;1000;1100;1200;1300;1400;1500;1600;1700;1800;1900;2000]  InternalRulePriority=Speed  RndMeth=Simplest
  Out1 : Outport
  wires:
  In1/1 -> LUT 0.98RR/1
  LUT 0.98RR/1 -> Out1/1

== system LUT_liver_pancreas_30/If Action Subsystem6/If Action Subsystem3/If Action Subsystem9/If Action Subsystem9 ==
  In1 : Inport
  Action Port : ActionPort  ActionPortLabel=if(u1 >= 0.985)
  LUT 0.99RR : Lookup_n-D  NumberOfTableDimensions=1  BreakpointsForDimension1=[466.5059;514.8482;613.3876;712.3848;811.3513;910.2534;1009.101;1107.905;1206.676;1305.421;1404.145;1502.849;1601.537;1700.207;1798.857;1897.476;1996.03]  Table=[400;500;600;700;800;900;1000;1100;1200;1300;1400;1500;1600;1700;1800;1900;2000]  InternalRulePriority=Speed  RndMeth=Simplest
  Out1 : Outport
  wires:
  In1/1 -> LUT 0.99RR/1
  LUT 0.99RR/1 -> Out1/1
